simulink model "lab_SF"  (R2021b)
settings: Solver=ode45  StartTime=0.0  StopTime=10.0  RelTol=1e-3
values from neighbouring files (symbols this model uses):
  A = [0, 1, 0, 0 ... (first row only)    [lab.m]
  B = [0 ... (first row only)    [lab.m]
  C = [1, 0, 0, 0 ... (first row only)    [lab.m]
  F = -acker(A, B, eign_F)    [lab.m]
  K = K2    [lab.m]
settings Model: Creator=ZIXUANXU  LastModifiedBy=gkbb
settings SolverCC: AlgebraicLoopSolver=TrustRegion
settings DataIOCC: ReturnWorkspaceOutputs=off  Refine=4
settings DebuggingCC: SFMachineParentedDataDiag=warning
settings SFSimCC: CustomCodeUndefinedFunction=UseInterfaceOnly

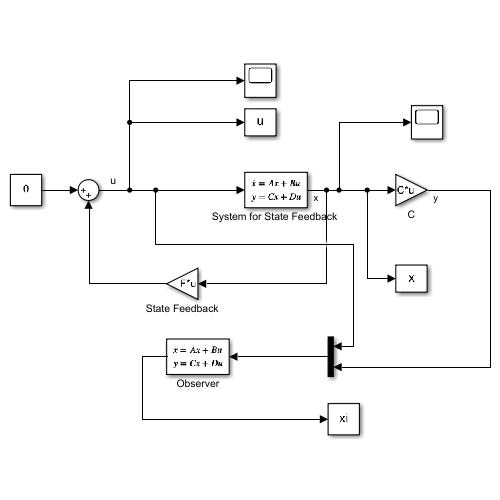
[thumbnail: Simulink's stored preview of the top-level diagram]
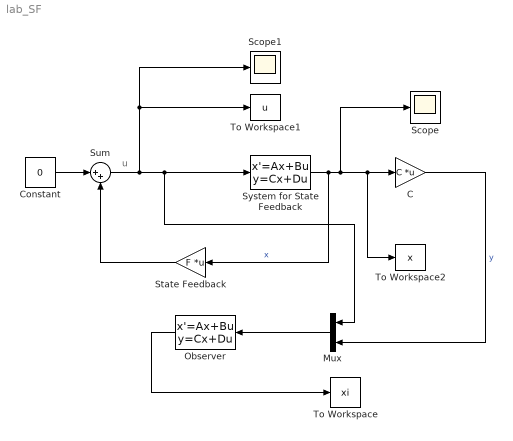
== system lab_SF ==
  note: u
  C : Gain  Gain=C  Multiplication=Matrix(K*u)
  Constant : Constant  Value=0
  Mux : Mux  Inputs=2
  Observer : StateSpace  A=[A - K*C]  B=[B K]  C=eye(4)  D=zeros(4, 3)  InitialCondition=[0 0 0 0]
  Scope : Scope
  Scope1 : Scope
  State Feedback : Gain  Gain=F  Multiplication=Matrix(K*u)
  Sum : Sum  Inputs=|++
  "System for State Feedback " : StateSpace  A=A  B=B  C=eye(4)  D=zeros(4,1)  InitialCondition=[0.1 0 0.1 0]
  To Workspace : ToWorkspace  VariableName=xi  SampleTime=-1
      settings: Save2DSignal=2-D array (concatenate along first dimension)
  To Workspace1 : ToWorkspace  VariableName=u  SampleTime=-1
      settings: Save2DSignal=2-D array (concatenate along first dimension)
  To Workspace2 : ToWorkspace  VariableName=x  SampleTime=-1
      settings: Save2DSignal=2-D array (concatenate along first dimension)
  wires:
  Constant/1 -> Sum/1
  Sum/1 -> To Workspace1/1, Scope1/1, Mux/1, "System for State Feedback "/1
  "System for State Feedback "/1 -> C/1, To Workspace2/1, Scope/1, State Feedback/1  "x"
  State Feedback/1 -> Sum/2
  Mux/1 -> Observer/1
  C/1 -> Mux/2  "y"
  Observer/1 -> To Workspace/1
